simulink model "Remus_pitch_control_PI_D_2022a"  (R2023b)
settings: Solver=ode1  StartTime=0.0  StopTime=T_final  FixedStep=Ts  RelTol=1e-3
values from neighbouring files (symbols this model uses):
  A = [-1.36757087013 -0.0298365607614 1.00305051334e-21 -2.85933126392 0.119442498277 -1.97014537421e-22 1 0 0 0 0 0 ... (144 elements, 12x12)]    [linmodel_u_2kts.mat]
  B = [0 -0.0899434384233 0 -0.353204156384 0 0.57859211058 0 0 0 0 0 0 ... (36 elements, 12x3)]    [linmodel_u_2kts.mat]
  C = [1 0 0 0 0 0 0 0 0 0 0 0 ... (144 elements, 12x12)]    [linmodel_u_2kts.mat]
  D = [0 0 0 0 0 0 0 0 0 0 0 0 ... (36 elements, 12x3)]    [linmodel_u_2kts.mat]
  Kd_theta = 0.115    [compare_PID.m]
  Ki_theta = 0.38    [compare_PID.m]
  Kp_theta = 0.6    [compare_PID.m]
  x0 = [2 -4.48954579629e-15 -5.26283161463e-21 1.99783697576e-20 -6.52845367291e-21 7.55477241533e-22 2.13618802829e-15 -1.75591256947e-16 1.82878054643e-16 0.109446709475 0 0]    [trim_u_2kts.mat]
settings Model: Creator=ADMIN  LastModifiedBy=admin
settings DebuggingCC: UnconnectedInputMsg=warning  UnconnectedOutputMsg=warning  UnconnectedLineMsg=warning
settings ModelReferenceCC: EnableRefExpFcnMdlSchedulingChecks=on
settings RTWCC: DLArmComputeVersion=19.05

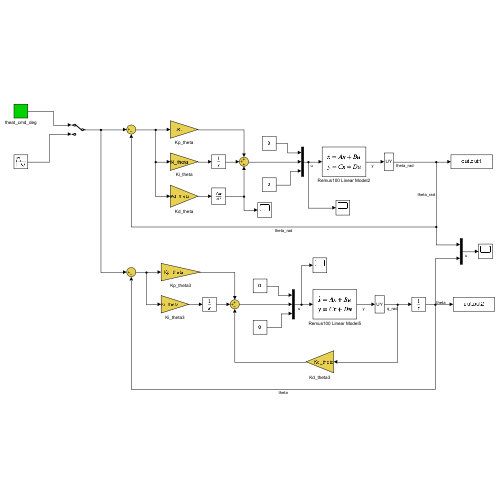
[thumbnail: Simulink's stored preview of the top-level diagram]
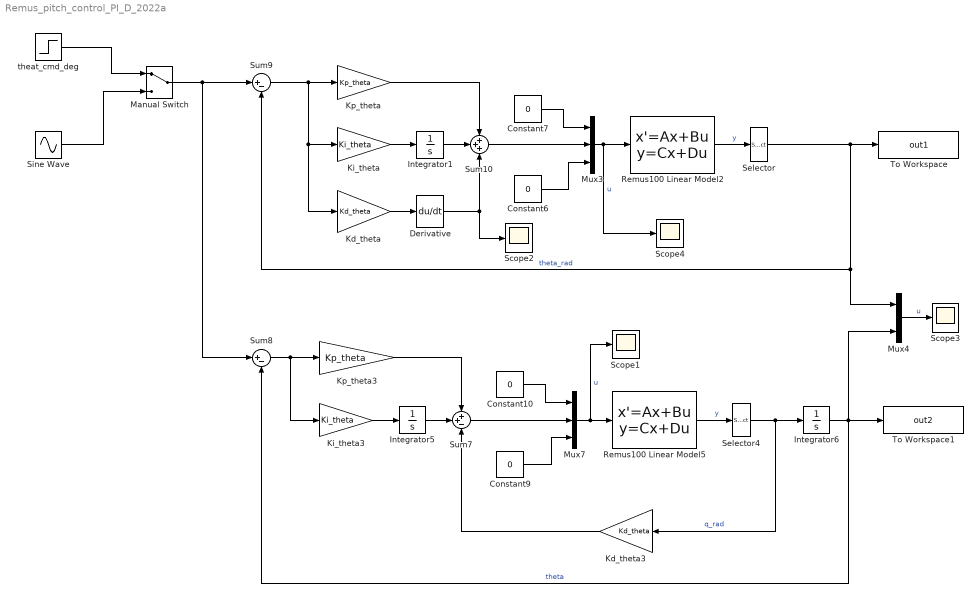
== system Remus_pitch_control_PI_D_2022a ==
  Constant{6..7,9..10} (4 alike) : Constant  Value=0  OutDataTypeStr=double
  Derivative : Derivative
  Integrator1 : Integrator
  Integrator5 : Integrator
  Integrator6 : Integrator
  Kd_theta : Gain  Gain=Kd_theta  SaturateOnIntegerOverflow=on  OutDataTypeStr=Inherit: Same as input  ParamDataTypeStr=Inherit: Same as input
  Kd_theta3 : Gain  Gain=Kd_theta  SaturateOnIntegerOverflow=on  OutDataTypeStr=Inherit: Same as input  ParamDataTypeStr=Inherit: Same as input
  Ki_theta : Gain  Gain=Ki_theta  SaturateOnIntegerOverflow=on  OutDataTypeStr=Inherit: Same as input  ParamDataTypeStr=Inherit: Same as input
  Ki_theta3 : Gain  Gain=Ki_theta  SaturateOnIntegerOverflow=on  OutDataTypeStr=Inherit: Same as input  ParamDataTypeStr=Inherit: Same as input
  Kp_theta : Gain  Gain=Kp_theta  SaturateOnIntegerOverflow=on  OutDataTypeStr=Inherit: Same as input  ParamDataTypeStr=Inherit: Same as input
  Kp_theta3 : Gain  Gain=Kp_theta  SaturateOnIntegerOverflow=on  OutDataTypeStr=Inherit: Same as input  ParamDataTypeStr=Inherit: Same as input
  Manual Switch : ManualSwitch
  Mux3 : Mux  Inputs=3
  Mux4 : Mux  Inputs=2
  Mux7 : Mux  Inputs=3
  Remus100 Linear Model2 : StateSpace  A=A  B=B  C=C  D=D  InitialCondition=x0*0
  Remus100 Linear Model5 : StateSpace  A=A  B=B  C=C  D=D  InitialCondition=x0*0
  Scope{1..4} (4 alike) : Scope
  Selector : Selector  InputPortWidth=12  IndexOptions=Index vector (dialog)  Indices=11  OutputSizes=1
  Selector4 : Selector  InputPortWidth=12  IndexOptions=Index vector (dialog)  Indices=5  OutputSizes=1
  Sine Wave : Sin  Frequency=20  SampleTime=0
  Sum10 : Sum  Inputs=+++  InputSameDT=on  SaturateOnIntegerOverflow=on  OutDataTypeStr=Inherit: Same as first input
  Sum7 : Sum  Inputs=++-  InputSameDT=on  SaturateOnIntegerOverflow=on  OutDataTypeStr=Inherit: Same as first input
  Sum8 : Sum  Inputs=|+-  InputSameDT=on  SaturateOnIntegerOverflow=on  OutDataTypeStr=Inherit: Same as first input
  Sum9 : Sum  Inputs=|+-  InputSameDT=on  SaturateOnIntegerOverflow=on  OutDataTypeStr=Inherit: Same as first input
  To Workspace : ToWorkspace  VariableName=out1  SaveFormat=Timeseries  SampleTime=-1
  To Workspace1 : ToWorkspace  VariableName=out2  SaveFormat=Timeseries  SampleTime=-1
  theat_cmd_deg : Step  SampleTime=0
  wires:
  Mux3/1 -> Scope4/1, Remus100 Linear Model2/1  "u"
  Constant6/1 -> Mux3/3
  Sum10/1 -> Mux3/2
  Constant7/1 -> Mux3/1
  Sum9/1 -> Kp_theta/1, Kd_theta/1, Ki_theta/1
  Selector/1 -> To Workspace/1, Mux4/1, Sum9/2  "theta_rad"
  Remus100 Linear Model2/1 -> Selector/1  "y"
  Integrator1/1 -> Sum10/2
  Kp_theta/1 -> Sum10/1
  Ki_theta/1 -> Integrator1/1
  Kd_theta/1 -> Derivative/1
  Derivative/1 -> Sum10/3, Scope2/1
  Mux4/1 -> Scope3/1  "u"
  Kd_theta3/1 -> Sum7/3
  Sum7/1 -> Mux7/2
  Manual Switch/1 -> Sum8/1, Sum9/1
  Kp_theta3/1 -> Sum7/1
  Ki_theta3/1 -> Integrator5/1
  Mux7/1 -> Scope1/1, Remus100 Linear Model5/1  "u"
  Sum8/1 -> Ki_theta3/1, Kp_theta3/1
  Constant10/1 -> Mux7/1
  Integrator5/1 -> Sum7/2
  Constant9/1 -> Mux7/3
  Remus100 Linear Model5/1 -> Selector4/1  "y"
  Selector4/1 -> Integrator6/1, Kd_theta3/1  "q_rad"
  Integrator6/1 -> To Workspace1/1, Mux4/2, Sum8/2  "theta"
  theat_cmd_deg/1 -> Manual Switch/1
  Sine Wave/1 -> Manual Switch/2
